simulink model "ERR_K5"  (R2025a)
settings: Solver=VariableStepAuto  StartTime=0.0  StopTime=500  MaxStep=0.1/25  RelTol=1e-3
libraries: simulink_extras x1
settings Model: Creator=Szalay  LastModifiedBy=Szalay

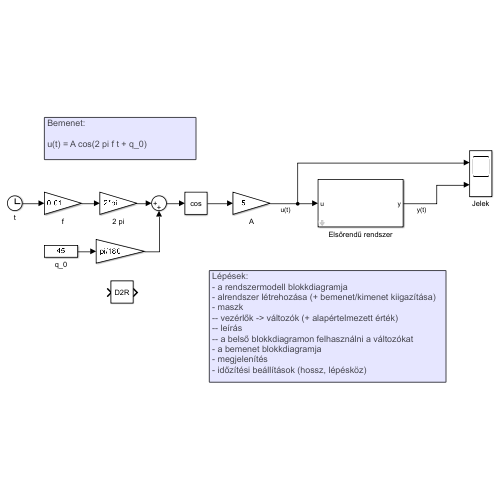
[thumbnail: Simulink's stored preview of the top-level diagram]
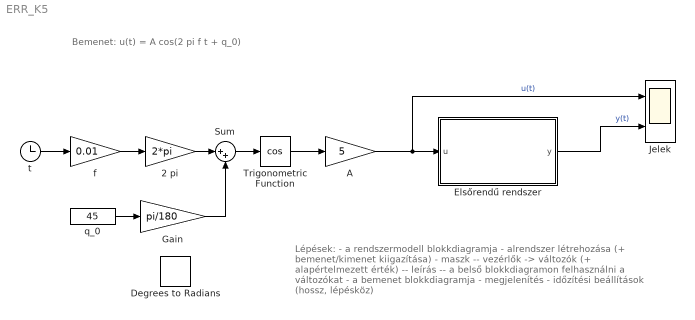
== system ERR_K5 ==
  note: Bemenet:
      |
      | u(t) = A cos(2 pi f t + q_0)
  note: Lépések:
      | - a rendszermodell blokkdiagramja
      | - alrendszer létrehozása (+ bemenet/kimenet kiigazítása)
      | - maszk
      | -- vezérlők -> változók (+ alapértelmezett érték)
      | -- leírás
      | -- a belső blokkdiagramon felhasználni a változókat
      | - a bemenet blokkdiagramja
      | - megjelenítés
      | - időzítési beállítások (hossz, lépésköz)
  2 pi : Gain  Gain=2*pi
  A : Gain  Gain=5
  Degrees to Radians : simulink_extras/Transformations/Degrees to Radians
  Elsőrendű rendszer : Subsystem  mask(Elsőrendű rendszer){K=1, tau=1, y_0=0}
      mask prompts: K "Állandósult állapoti erősítés"; tau "Időállandó (s)"; y_0 "Kezdeti érték"
      mask help: A lineáris elsőrendű rendszer modellje.
      mask DialogControl ParameterGroupVar Prompt: Modellparaméterek
      mask DialogControl Container3 Prompt: Kezdeti érték
  Gain : Gain  Gain=pi/180
  Jelek : Scope  NumInputPorts=2
      settings: ActiveDisplayYMinimum=-6.2376993926082385  ActiveDisplayYMaximum=6.2376993926082358
  Sum : Sum  Inputs=|++
  Trigonometric Function : Trigonometry  Operator=cos
  f : Gain  Gain=0.01
  q_0 : Constant  Value=45
  t : Clock
  wires:
  A/1 -> Jelek/1, Elsőrendű rendszer/1(u)  "u(t)"
  Trigonometric Function/1 -> A/1
  Sum/1 -> Trigonometric Function/1
  q_0/1 -> Gain/1
  Gain/1 -> Sum/2
  2 pi/1 -> Sum/1
  f/1 -> 2 pi/1
  t/1 -> f/1
  Elsőrendű rendszer/1(y) -> Jelek/2  "y(t)"

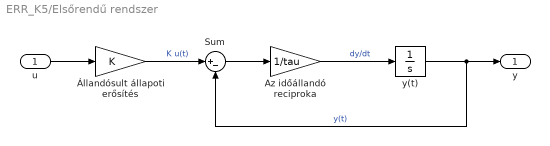
== system ERR_K5/Elsőrendű rendszer ==
  u : Inport
  Az időállandó reciproka : Gain  Gain=1/tau
  Sum : Sum  Inputs=|+-
  y(t) : Integrator  InitialCondition=y_0
  Állandósult állapoti erősítés : Gain  Gain=K
  y : Outport
  wires:
  y(t)/1 -> y/1, Sum/2  "y(t)"
  u/1 -> Állandósult állapoti erősítés/1
  Sum/1 -> Az időállandó reciproka/1
  Állandósult állapoti erősítés/1 -> Sum/1  "K u(t)"
  Az időállandó reciproka/1 -> y(t)/1  "dy/dt"
